simulink model "estimator_designs_main"  (R2022b)
settings: Solver=ode4  StartTime=0.0  StopTime=T  FixedStep=0.002  RelTol=1e-3
values from neighbouring files (symbols this model uses):
  c_lat_f = u(11)    [modelBasedSpeedEstForKalman.m]    (also in validation.m = 140000)
  c_lat_r = u(12)    [modelBasedSpeedEstForKalman.m]    (also in validation.m = 150000)
  c_lon_f = u(9)    [modelBasedSpeedEstForKalman.m]    (also in validation.m = 180000)
  c_lon_r = u(10)    [modelBasedSpeedEstForKalman.m]    (also in validation.m = 200000)
  dt = u(4)    [kinematicVelocity.m]    (also in modelBasedSpeedEstForKalman.m = u(27); validation.m = 0.01)
  eps_bw_acc = 0.1    [validation.m]
  eps_ekf_m_bw_v_u = 0.5    [validation.m]
  eps_m_v = 1    [validation.m]
  m = u(7)    [modelBasedSpeedEstForKalman.m]    (also in validation.m = 3020)
  num_of_signals = 12    [validation.m]
  P0 = diag([1e-5, 1e-5, 1e-5])    [validation.m]
  Q_ekf_1 = diag([1e-5, 1e-2, 1e-2])    [validation.m]
  R = u(9)    [bestWheelSpeedUpdate.m]    (also in modelBasedSpeedEstForKalman.m = u(13); validation.m = 0.3615)
  r_COG_FL = u(10:12)    [bestWheelSpeedUpdate.m]    (also in validation.m = [wheelbase_COG_front; front_track_width / 2; 0])
  r_COG_FR = u(13:15)    [bestWheelSpeedUpdate.m]    (also in validation.m = [wheelbase_COG_front; -front_track_width / 2; 0])
  r_COG_RL = u(16:18)    [bestWheelSpeedUpdate.m]    (also in validation.m = [-wheelbase_COG_rear; rear_track_width / 2; 0])
  r_COG_RR = u(19:21)    [bestWheelSpeedUpdate.m]    (also in validation.m = [-wheelbase_COG_rear; -rear_track_width / 2; 0])
  R_ekf_1 = 1e-2    (= 0.01)    [validation.m]
  sequence_length = 50    [validation.m]
  theta_z = 7145    [validation.m]
  thr_ekf_m_bw_v_u = 5    [validation.m]
  x0 = [0.0001; 0.0001; 0.0001]    [validation.m]
undefined symbols (not defined in the file or in its folder): Discrete, Time
libraries: deeplib x2, ctrlSharedLib x1
(part 1 of 2)
settings Model: Creator=andrzej.skrodzki  LastModifiedBy=andrzej.skrodzki
settings DebuggingCC: SignalInfNanChecking=error  AlgebraicLoopMsg=error  CheckMatrixSingularityMsg=error  IntegerOverflowMsg=error  UnnecessaryDatatypeConvMsg=warning  SignalLabelMismatchMsg=warning  UnconnectedInputMsg=warning  UnconnectedOutputMsg=warning  UnconnectedLineMsg=warning  StrictBusMsg=ErrorOnBusTreatedAsVector  IntegerSaturationMsg=error

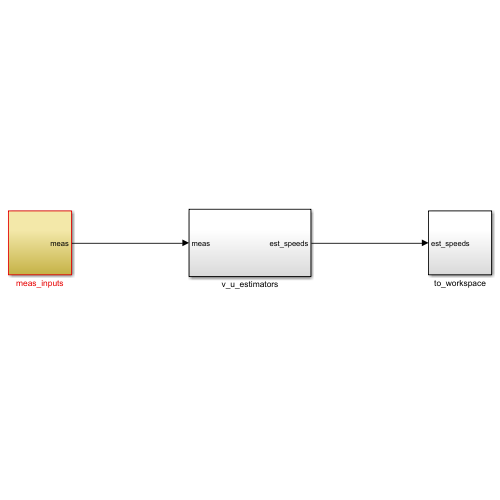
[thumbnail: Simulink's stored preview of the top-level diagram]
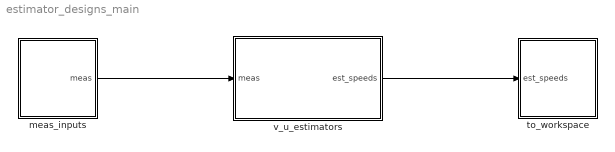
== system estimator_designs_main ==
  meas_inputs : Subsystem
  to_workspace : Subsystem
  v_u_estimators : Subsystem
  wires:
  meas_inputs/1(meas) -> v_u_estimators/1(meas)
  v_u_estimators/1(est_speeds) -> to_workspace/1(est_speeds)

== system estimator_designs_main/meas_inputs ==
  Rate Transition : RateTransition  OutPortSampleTime=0.01
  measurement_replay : Subsystem
  parameters : Subsystem
  sequence_generator : Subsystem
  Bus Element Out : Outport  PortName=meas  Element=SENS_IN_ai_seq_t
  Bus Element Out1 : Outport  PortName=meas  Element=SENS_IN_ai_seq_inf
  Bus Element Out2 : Outport  PortName=meas  Element=SENS_IN
  Bus Element Out3 : Outport  PortName=meas  Element=params
  wires:
  sequence_generator/2(SENS_IN_ai_seq_inf) -> Bus Element Out1/1  "SENS_IN_ai_seq_inf"
  sequence_generator/1(SENS_IN_ai_seq_t) -> Bus Element Out/1  "SENS_IN_ai_seq_t"
  Rate Transition/1 -> Bus Element Out2/1  "SENS_IN"
  measurement_replay/1(SENS_IN) -> Rate Transition/1
  parameters/1(params) -> Bus Element Out3/1

== system estimator_designs_main/to_workspace ==
  BusElementIn : Inport  PortName=est_speeds  Element=v_u_bw
  BusElementIn1 : Inport  PortName=est_speeds  Element=v_u_m
  BusElementIn2 : Inport  PortName=est_speeds  Element=v_u_ekf_m_bw
  BusElementIn3 : Inport  PortName=est_speeds  Element=v_u_ekf_m_ai
  BusElementIn4 : Inport  PortName=est_speeds  Element=veh_u_i7
  BusElementIn5 : Inport  PortName=est_speeds  Element=veh_v
  BusElementIn6 : Inport  PortName=est_speeds  Element=veh_u
  To Workspace : ToWorkspace  VariableName=model_based  SaveFormat=Timeseries  SampleTime=-1
  To Workspace1 : ToWorkspace  VariableName=best_wheel  SaveFormat=Timeseries  SampleTime=-1
  To Workspace2 : ToWorkspace  VariableName=veh_ref  SaveFormat=Timeseries  SampleTime=-1
  To Workspace3 : ToWorkspace  VariableName=ekf_m_bw  SaveFormat=Timeseries  SampleTime=-1
  To Workspace4 : ToWorkspace  VariableName=veh_u  SaveFormat=Timeseries  SampleTime=-1
  To Workspace5 : ToWorkspace  VariableName=veh_v  SaveFormat=Timeseries  SampleTime=-1
  To Workspace6 : ToWorkspace  VariableName=ekf_ai  SaveFormat=Timeseries  SampleTime=-1
  wires:
  BusElementIn4/1 -> To Workspace2/1
  BusElementIn2/1 -> To Workspace3/1
  BusElementIn/1 -> To Workspace1/1
  BusElementIn5/1 -> To Workspace4/1
  BusElementIn3/1 -> To Workspace6/1
  BusElementIn6/1 -> To Workspace5/1
  BusElementIn1/1 -> To Workspace/1

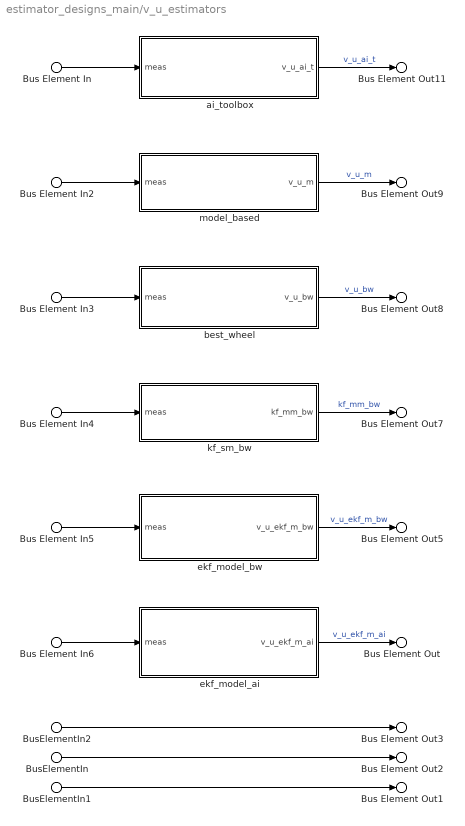
== system estimator_designs_main/v_u_estimators ==
  Bus Element In{,2..6} (6 alike) : Inport  PortName=meas
  BusElementIn : Inport  PortName=meas  Element=SENS_IN.veh_u
  BusElementIn1 : Inport  PortName=meas  Element=SENS_IN.veh_v
  BusElementIn2 : Inport  PortName=meas  Element=SENS_IN.veh_u_i7
  ai_toolbox : Subsystem
  best_wheel : Subsystem
  ekf_model_ai : Subsystem
  ekf_model_bw : Subsystem
  kf_sm_bw : Subsystem
  model_based : Subsystem
  Bus Element Out : Outport  PortName=est_speeds  Element=v_u_ekf_m_ai
  Bus Element Out1 : Outport  PortName=est_speeds  Element=veh_v
  Bus Element Out2 : Outport  PortName=est_speeds  Element=veh_u
  Bus Element Out3 : Outport  PortName=est_speeds  Element=veh_u_i7
  Bus Element Out5 : Outport  PortName=est_speeds  Element=v_u_ekf_m_bw
  Bus Element Out7 : Outport  PortName=est_speeds  Element=v_u_kf_mm_bw
  Bus Element Out8 : Outport  PortName=est_speeds  Element=v_u_bw
  Bus Element Out9 : Outport  PortName=est_speeds  Element=v_u_m
  Bus Element Out11 : Outport  PortName=est_speeds  Element=v_u_ai_t
  wires:
  model_based/1(v_u_m) -> Bus Element Out9/1  "v_u_m"
  best_wheel/1(v_u_bw) -> Bus Element Out8/1  "v_u_bw"
  BusElementIn/1 -> Bus Element Out2/1
  ekf_model_bw/1(v_u_ekf_m_bw) -> Bus Element Out5/1  "v_u_ekf_m_bw"
  ekf_model_ai/1(v_u_ekf_m_ai) -> Bus Element Out/1  "v_u_ekf_m_ai"
  ai_toolbox/1(v_u_ai_t) -> Bus Element Out11/1  "v_u_ai_t"
  kf_sm_bw/1(kf_mm_bw) -> Bus Element Out7/1  "kf_mm_bw"
  BusElementIn1/1 -> Bus Element Out1/1
  BusElementIn2/1 -> Bus Element Out3/1
  Bus Element In/1 -> ai_toolbox/1(meas)
  Bus Element In6/1 -> ekf_model_ai/1(meas)
  Bus Element In5/1 -> ekf_model_bw/1(meas)
  Bus Element In4/1 -> kf_sm_bw/1(meas)
  Bus Element In3/1 -> best_wheel/1(meas)
  Bus Element In2/1 -> model_based/1(meas)

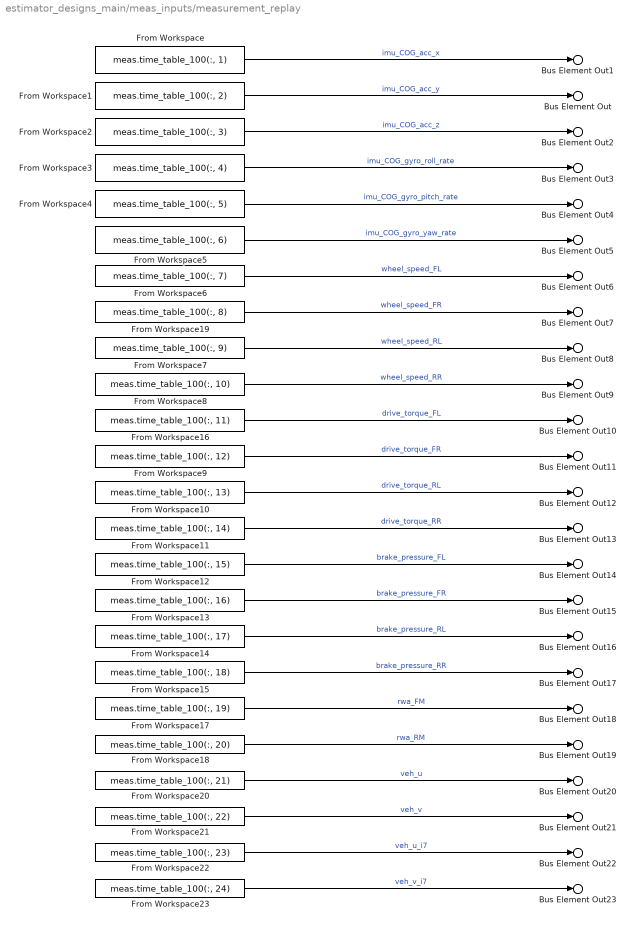
== system estimator_designs_main/meas_inputs/measurement_replay ==
  From Workspace : FromWorkspace  VariableName=meas.time_table_100(:, 1)
  From Workspace1 : FromWorkspace  VariableName=meas.time_table_100(:, 2)
  From Workspace10 : FromWorkspace  VariableName=meas.time_table_100(:, 13)
  From Workspace11 : FromWorkspace  VariableName=meas.time_table_100(:, 14)
  From Workspace12 : FromWorkspace  VariableName=meas.time_table_100(:, 15)
  From Workspace13 : FromWorkspace  VariableName=meas.time_table_100(:, 16)
  From Workspace14 : FromWorkspace  VariableName=meas.time_table_100(:, 17)
  From Workspace15 : FromWorkspace  VariableName=meas.time_table_100(:, 18)
  From Workspace16 : FromWorkspace  VariableName=meas.time_table_100(:, 11)
  From Workspace17 : FromWorkspace  VariableName=meas.time_table_100(:, 19)
  From Workspace18 : FromWorkspace  VariableName=meas.time_table_100(:, 20)
  From Workspace19 : FromWorkspace  VariableName=meas.time_table_100(:, 8)
  From Workspace2 : FromWorkspace  VariableName=meas.time_table_100(:, 3)
  From Workspace20 : FromWorkspace  VariableName=meas.time_table_100(:, 21)
  From Workspace21 : FromWorkspace  VariableName=meas.time_table_100(:, 22)
  From Workspace22 : FromWorkspace  VariableName=meas.time_table_100(:, 23)
  From Workspace23 : FromWorkspace  VariableName=meas.time_table_100(:, 24)
  From Workspace3 : FromWorkspace  VariableName=meas.time_table_100(:, 4)
  From Workspace4 : FromWorkspace  VariableName=meas.time_table_100(:, 5)
  From Workspace5 : FromWorkspace  VariableName=meas.time_table_100(:, 6)
  From Workspace6 : FromWorkspace  VariableName=meas.time_table_100(:, 7)
  From Workspace7 : FromWorkspace  VariableName=meas.time_table_100(:, 9)
  From Workspace8 : FromWorkspace  VariableName=meas.time_table_100(:, 10)
  From Workspace9 : FromWorkspace  VariableName=meas.time_table_100(:, 12)
  Bus Element Out : Outport  PortName=SENS_IN  Element=imu_COG_acc_y
  Bus Element Out1 : Outport  PortName=SENS_IN  Element=imu_COG_acc_x
  Bus Element Out2 : Outport  PortName=SENS_IN  Element=imu_COG_acc_z
  Bus Element Out3 : Outport  PortName=SENS_IN  Element=imu_COG_gyro_roll_rate
  Bus Element Out4 : Outport  PortName=SENS_IN  Element=imu_COG_gyro_pitch_rate
  Bus Element Out5 : Outport  PortName=SENS_IN  Element=imu_COG_gyro_yaw_rate
  Bus Element Out6 : Outport  PortName=SENS_IN  Element=wheel_speed_FL
  Bus Element Out7 : Outport  PortName=SENS_IN  Element=wheel_speed_FR
  Bus Element Out8 : Outport  PortName=SENS_IN  Element=wheel_speed_RL
  Bus Element Out9 : Outport  PortName=SENS_IN  Element=wheel_speed_RR
  Bus Element Out10 : Outport  PortName=SENS_IN  Element=drive_torque_FL
  Bus Element Out11 : Outport  PortName=SENS_IN  Element=drive_torque_FR
  Bus Element Out12 : Outport  PortName=SENS_IN  Element=drive_torque_RL
  Bus Element Out13 : Outport  PortName=SENS_IN  Element=drive_torque_RR
  Bus Element Out14 : Outport  PortName=SENS_IN  Element=brake_pressure_FL
  Bus Element Out15 : Outport  PortName=SENS_IN  Element=brake_pressure_FR
  Bus Element Out16 : Outport  PortName=SENS_IN  Element=brake_pressure_RL
  Bus Element Out17 : Outport  PortName=SENS_IN  Element=brake_pressure_RR
  Bus Element Out18 : Outport  PortName=SENS_IN  Element=rwa_FM
  Bus Element Out19 : Outport  PortName=SENS_IN  Element=rwa_RM
  Bus Element Out20 : Outport  PortName=SENS_IN  Element=veh_u
  Bus Element Out21 : Outport  PortName=SENS_IN  Element=veh_v
  Bus Element Out22 : Outport  PortName=SENS_IN  Element=veh_u_i7
  Bus Element Out23 : Outport  PortName=SENS_IN  Element=veh_v_i7
  wires:
  From Workspace5/1 -> Bus Element Out5/1  "imu_COG_gyro_yaw_rate"
  From Workspace8/1 -> Bus Element Out9/1  "wheel_speed_RR"
  From Workspace17/1 -> Bus Element Out18/1  "rwa_FM"
  From Workspace18/1 -> Bus Element Out19/1  "rwa_RM"
  From Workspace4/1 -> Bus Element Out4/1  "imu_COG_gyro_pitch_rate"
  From Workspace19/1 -> Bus Element Out7/1  "wheel_speed_FR"
  From Workspace6/1 -> Bus Element Out6/1  "wheel_speed_FL"
  From Workspace15/1 -> Bus Element Out17/1  "brake_pressure_RR"
  From Workspace16/1 -> Bus Element Out10/1  "drive_torque_FL"
  From Workspace3/1 -> Bus Element Out3/1  "imu_COG_gyro_roll_rate"
  From Workspace12/1 -> Bus Element Out14/1  "brake_pressure_FL"
  From Workspace2/1 -> Bus Element Out2/1  "imu_COG_acc_z"
  From Workspace10/1 -> Bus Element Out12/1  "drive_torque_RL"
  From Workspace11/1 -> Bus Element Out13/1  "drive_torque_RR"
  From Workspace14/1 -> Bus Element Out16/1  "brake_pressure_RL"
  From Workspace7/1 -> Bus Element Out8/1  "wheel_speed_RL"
  From Workspace13/1 -> Bus Element Out15/1  "brake_pressure_FR"
  From Workspace1/1 -> Bus Element Out/1  "imu_COG_acc_y"
  From Workspace9/1 -> Bus Element Out11/1  "drive_torque_FR"
  From Workspace/1 -> Bus Element Out1/1  "imu_COG_acc_x"
  From Workspace20/1 -> Bus Element Out20/1  "veh_u"
  From Workspace21/1 -> Bus Element Out21/1  "veh_v"
  From Workspace22/1 -> Bus Element Out22/1  "veh_u_i7"
  From Workspace23/1 -> Bus Element Out23/1  "veh_v_i7"

== system estimator_designs_main/meas_inputs/parameters ==
  constants : Subsystem
  Bus Element Out : Outport  PortName=params  Element=m
  Bus Element Out1 : Outport  PortName=params  Element=I_z
  Bus Element Out2 : Outport  PortName=params  Element=C
  Bus Element Out3 : Outport  PortName=params  Element=R
  Bus Element Out4 : Outport  PortName=params  Element=r
  Bus Element Out5 : Outport  PortName=params  Element=eps_m_v
  Bus Element Out6 : Outport  PortName=params  Element=dt
  Bus Element Out7 : Outport  PortName=params  Element=eps_bw_acc
  Bus Element Out8 : Outport  PortName=params  Element=thr_ekf_m_bw_v_u
  Bus Element Out9 : Outport  PortName=params  Element=eps_ekf_m_bw_v_u
  Bus Element Out10 : Outport  PortName=params  Element=R_ekf_1
  Bus Element Out11 : Outport  PortName=params  Element=Q_ekf_1
  wires:
  constants/1(m) -> Bus Element Out/1
  constants/2(I_z) -> Bus Element Out1/1
  constants/3(C) -> Bus Element Out2/1
  constants/4(R) -> Bus Element Out3/1
  constants/5(r) -> Bus Element Out4/1
  constants/6(eps_m_v) -> Bus Element Out5/1
  constants/7(dt) -> Bus Element Out6/1
  constants/8(eps_bw_acc) -> Bus Element Out7/1
  constants/9(thr_ekf_m_bw_v_u) -> Bus Element Out8/1
  constants/10(eps_ekf_m_bw_v_u) -> Bus Element Out9/1
  constants/11(R_ekf_1) -> Bus Element Out10/1
  constants/12(Q_ekf_1) -> Bus Element Out11/1

== system estimator_designs_main/meas_inputs/sequence_generator ==
  Constant1 : Constant  Value=zeros(num_of_signals, sequence_length)
  Constant2 : Constant  Value=zeros(sequence_length, num_of_signals)
  Delay1 : Delay  DelayLength=1  InitialConditionSource=Input port
      settings: InputPortMap=u0,p4
  Delay2 : Delay  DelayLength=1  InitialConditionSource=Input port
      settings: InputPortMap=u0,p4
  MATLAB Function1 : MATLAB Function  TreatAsAtomicUnit=on
  MATLAB Function4 : MATLAB Function  TreatAsAtomicUnit=on
  Rate Transition1 : RateTransition  OutPortSampleTime=0.01
  Reshape : Reshape  OutputDimensionality=Customize  OutputDimensions=[1, sequence_length, num_of_signals]
  Subsystem : Subsystem
  SENS_IN_ai_seq_t : Outport
  SENS_IN_ai_seq_inf : Outport  Port=2
  wires:
  Rate Transition1/1 -> MATLAB Function4/1(SNES_IN_ai), MATLAB Function1/1(SENS_IN_ai)  "SENS_IN_ai"
  Reshape/1 -> SENS_IN_ai_seq_inf/1  "SENS_IN_ai_seq_inf"
  MATLAB Function4/1(SENS_IN_ai_seq) -> Delay2/1, Reshape/1  "SNES_IN_ai_seq_inf"
  Subsystem/1(SENS_IN_ai) -> Rate Transition1/1
  Delay2/1 -> MATLAB Function4/2(SENS_IN_ai_seq_prev)
  Constant2/1 -> Delay2/2
  Constant1/1 -> Delay1/2
  MATLAB Function1/1(SENS_IN_ai_seq) -> SENS_IN_ai_seq_t/1, Delay1/1  "SENS_IN_ai_seq_t"
  Delay1/1 -> MATLAB Function1/2(SENS_IN_ai_seq_prev)

== system estimator_designs_main/v_u_estimators/ai_toolbox ==
  BusElementIn : Inport  PortName=meas  Element=SENS_IN_ai_seq_t
  Reshape : Reshape  Commented=on  OutputDimensionality=Customize  OutputDimensions=[1,sequence_length, num_of_signals]
  "built-in ai " : deeplib/Predict  Network=Network from MAT-file  NetworkFunction=squeezenet  NetworkFilePath=file:///C:/work/0_currently_in_use/AI_training_matlab/trained_models/GRU/trainedGRU.mat  MiniBatchSize=1  InputDataFormats={'',''}  Predictions=on  Activations={}  ForceInterpretedSim=off  EnableDLNetwork=on
  built-in ai 1 : deeplib/Predict  Commented=on  Network=Network from MAT-file  NetworkFunction=squeezenet  NetworkFilePath=file:///C:/work/0_currently_in_use/estimator_designs/models/TCN/it_1/for_matlab/mat/lon/model_TCN_lon 129_conv2d.mat  MiniBatchSize=1  InputDataFormats={ 'input', 'BTC' }  Predictions=on  Activations={}  ForceInterpretedSim=off  EnableDLNetwork=on
  v_u_ai_t : Outport
  wires:
  BusElementIn/1 -> Reshape/1, "built-in ai "/1
  "built-in ai "/1 -> v_u_ai_t/1  "v_u_ai_t"
  built-in ai 1/1 -> ?  "v_u_ai_t"
  Reshape/1 -> built-in ai 1/1

== system estimator_designs_main/v_u_estimators/best_wheel ==
  meas : Inport
  Delay : Delay  DelayLength=1
  best_wheel_speed_est : MATLAB Function  TreatAsAtomicUnit=on
  input_generator : Subsystem
  v_u_bw : Outport
  wires:
  best_wheel_speed_est/1(v_u_bw) -> v_u_bw/1  "v_u_bw"
  meas/1 -> input_generator/1(meas)
  input_generator/1(u) -> best_wheel_speed_est/1(u)
  best_wheel_speed_est/2(sign_acc) -> Delay/1
  Delay/1 -> input_generator/2(prev_sign_acc)

== system estimator_designs_main/v_u_estimators/ekf_model_ai ==
  meas : Inport
  ai_inference_function : Subsystem
  ekf_custom : Subsystem
  input_generator_model : Subsystem
  v_u_ekf_m_ai : Outport
  wires:
  input_generator_model/1(StateTransitionFcnInputs) -> ekf_custom/1(StateTransitionFcnInputs)
  meas/1 -> ekf_custom/3(meas), ai_inference_function/1(meas), input_generator_model/1(meas)
  ai_inference_function/1(v_u_ai_inf) -> ekf_custom/2(v_u_ai_inf)
  ekf_custom/1(v_u_ekf_m_bw) -> v_u_ekf_m_ai/1  "v_u_ekf_m_ai"

== system estimator_designs_main/v_u_estimators/ekf_model_bw ==
  meas : Inport
  ekf_custom : Subsystem
  input_generator_model : Subsystem
  meas_update_bw : Subsystem
  v_u_ekf_m_bw : Outport
  wires:
  meas/1 -> ekf_custom/3(meas), meas_update_bw/1(meas), input_generator_model/1(meas)
  input_generator_model/1(StateTransitionFcnInputs) -> ekf_custom/1(StateTransitionFcnInputs)
  meas_update_bw/1(v_u_bw) -> ekf_custom/2(v_u_bw)
  ekf_custom/1(v_u_ekf_m_bw) -> v_u_ekf_m_bw/1  "v_u_ekf_m_bw"

== system estimator_designs_main/v_u_estimators/kf_sm_bw ==
  meas : Inport
  Selector1 : Selector  InputPortWidth=3  IndexOptions=Index vector (dialog)  Indices=[1]  OutputSizes=1
  Terminator : Terminator
  kf_sm : ctrlSharedLib/Kalman Filter  TimeDomain=Discrete-Time  UseCurrentEstimator=on  ModelSource=Individual A, B, C, D matrices  ModelSourceVariable=ss(0.95,1,1,0,1)  A=diag([1, 0.99, 0.99])  B=0  C=[1,0,0]  D=0  NumberOfStates=1  NumberOfInputs=1  NumberOfOutputs=1  InitialEstimateSource=Dialog  X0=[0;0;0]  P0=10  UseK=off  UseGH=off  NumberOfProcessNoiseInputs=1  G=1  TimeInvariantG=on  H=0  TimeInvariantH=on  Q=diag([0.0025, 0.04, 7.615e-5])  TimeInvariantQ=on  R=0.001  TimeInvariantR=on  N=0  TimeInvariantN=on  AddInputPort=off  AddEnablePort=off  OutputEstimatedY=off  OutputP=off  Ts=-1
  meas_update_ai : Subsystem
  meas_update_bw : Subsystem
  kf_mm_bw : Outport
  wires:
  kf_sm/1 -> Selector1/1
  Selector1/1 -> kf_mm_bw/1
  meas_update_bw/1(v_u_bw) -> kf_sm/1
  meas/1 -> meas_update_ai/1(meas), meas_update_bw/1(meas)
  meas_update_ai/1(v_u_ai_inf) -> Terminator/1

== system estimator_designs_main/v_u_estimators/model_based ==
  meas : Inport
  Delay : Delay  DelayLength=1
  Selector : Selector  InputPortWidth=3  IndexOptions=Index vector (dialog)  Indices=[1]  OutputSizes=1
  input_generator : Subsystem
  model_based_speed_est1 : MATLAB Function  TreatAsAtomicUnit=on
  v_u_m : Outport
  wires:
  model_based_speed_est1/1(x_plus) -> Selector/1, Delay/1  "x_plus"
  Delay/1 -> model_based_speed_est1/1(x)
  meas/1 -> input_generator/1(meas)
  input_generator/1(u) -> model_based_speed_est1/2(u)
  Selector/1 -> v_u_m/1  "v_u_m"

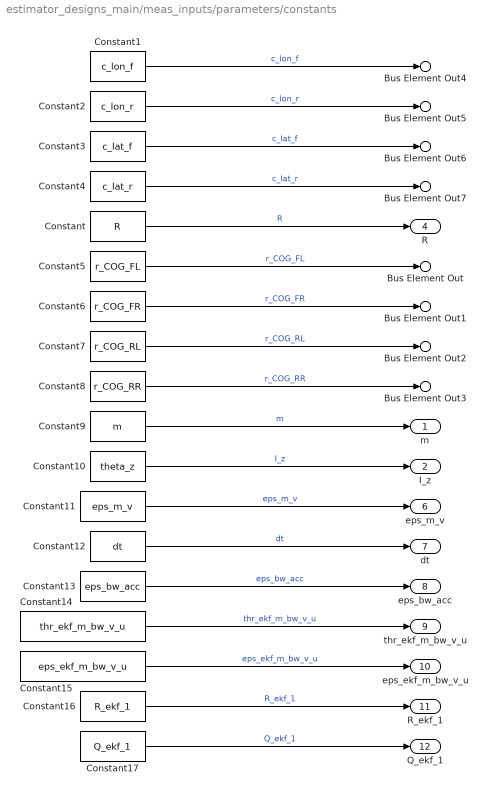
== system estimator_designs_main/meas_inputs/parameters/constants ==
  Constant : Constant  Value=R
  Constant1 : Constant  Value=c_lon_f
  Constant10 : Constant  Value=theta_z
  Constant11 : Constant  Value=eps_m_v
  Constant12 : Constant  Value=dt
  Constant13 : Constant  Value=eps_bw_acc
  Constant14 : Constant  Value=thr_ekf_m_bw_v_u
  Constant15 : Constant  Value=eps_ekf_m_bw_v_u
  Constant16 : Constant  Value=R_ekf_1
  Constant17 : Constant  Value=Q_ekf_1
  Constant2 : Constant  Value=c_lon_r
  Constant3 : Constant  Value=c_lat_f
  Constant4 : Constant  Value=c_lat_r
  Constant5 : Constant  Value=r_COG_FL
  Constant6 : Constant  Value=r_COG_FR
  Constant7 : Constant  Value=r_COG_RL
  Constant8 : Constant  Value=r_COG_RR
  Constant9 : Constant  Value=m
  m : Outport
  I_z : Outport  Port=2
  Bus Element Out4 : Outport  Port=3  PortName=C  Element=c_lon_f
  Bus Element Out5 : Outport  Port=3  PortName=C  Element=c_lon_r
  Bus Element Out6 : Outport  Port=3  PortName=C  Element=c_lat_f
  Bus Element Out7 : Outport  Port=3  PortName=C  Element=c_lat_r
  R : Outport  Port=4
  Bus Element Out : Outport  Port=5  PortName=r  Element=r_COG_FL
  Bus Element Out1 : Outport  Port=5  PortName=r  Element=r_COG_FR
  Bus Element Out2 : Outport  Port=5  PortName=r  Element=r_COG_RL
  Bus Element Out3 : Outport  Port=5  PortName=r  Element=r_COG_RR
  eps_m_v : Outport  Port=6
  dt : Outport  Port=7
  eps_bw_acc : Outport  Port=8
  thr_ekf_m_bw_v_u : Outport  Port=9
  eps_ekf_m_bw_v_u : Outport  Port=10
  R_ekf_1 : Outport  Port=11
  Q_ekf_1 : Outport  Port=12
  wires:
  Constant6/1 -> Bus Element Out1/1  "r_COG_FR"
  Constant3/1 -> Bus Element Out6/1  "c_lat_f"
  Constant4/1 -> Bus Element Out7/1  "c_lat_r"
  Constant/1 -> R/1  "R"
  Constant7/1 -> Bus Element Out2/1  "r_COG_RL"
  Constant1/1 -> Bus Element Out4/1  "c_lon_f"
  Constant5/1 -> Bus Element Out/1  "r_COG_FL"
  Constant8/1 -> Bus Element Out3/1  "r_COG_RR"
  Constant2/1 -> Bus Element Out5/1  "c_lon_r"
  Constant9/1 -> m/1  "m"
  Constant10/1 -> I_z/1  "I_z"
  Constant11/1 -> eps_m_v/1  "eps_m_v"
  Constant12/1 -> dt/1  "dt"
  Constant13/1 -> eps_bw_acc/1  "eps_bw_acc"
  Constant14/1 -> thr_ekf_m_bw_v_u/1  "thr_ekf_m_bw_v_u"
  Constant15/1 -> eps_ekf_m_bw_v_u/1  "eps_ekf_m_bw_v_u"
  Constant16/1 -> R_ekf_1/1  "R_ekf_1"
  Constant17/1 -> Q_ekf_1/1  "Q_ekf_1"

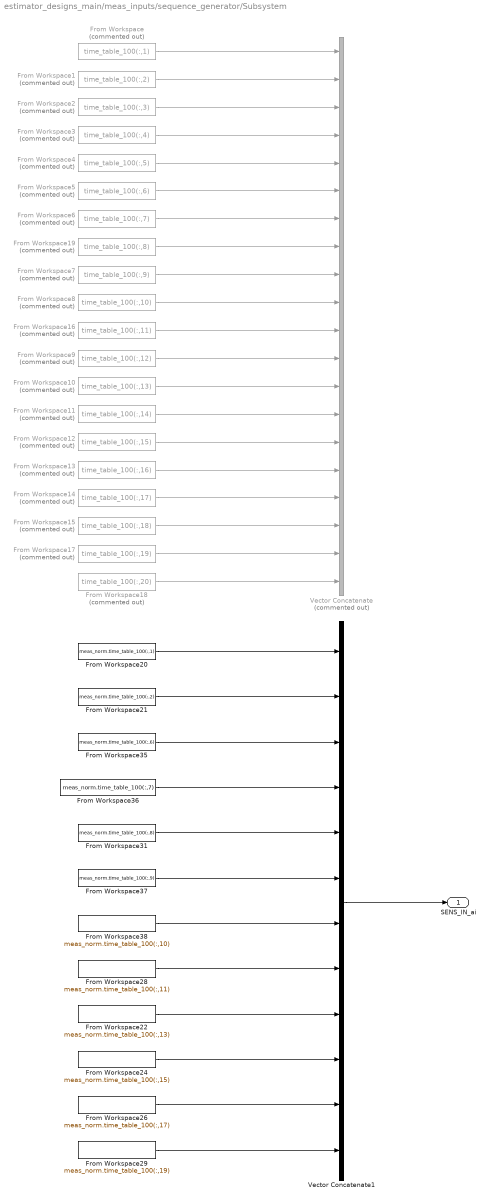
== system estimator_designs_main/meas_inputs/sequence_generator/Subsystem ==
  From Workspace : FromWorkspace  Commented=on  VariableName=time_table_100(:,1)
  From Workspace1 : FromWorkspace  Commented=on  VariableName=time_table_100(:,2)
  From Workspace10 : FromWorkspace  Commented=on  VariableName=time_table_100(:,13)
  From Workspace11 : FromWorkspace  Commented=on  VariableName=time_table_100(:,14)
  From Workspace12 : FromWorkspace  Commented=on  VariableName=time_table_100(:,15)
  From Workspace13 : FromWorkspace  Commented=on  VariableName=time_table_100(:,16)
  From Workspace14 : FromWorkspace  Commented=on  VariableName=time_table_100(:,17)
  From Workspace15 : FromWorkspace  Commented=on  VariableName=time_table_100(:,18)
  From Workspace16 : FromWorkspace  Commented=on  VariableName=time_table_100(:,11)
  From Workspace17 : FromWorkspace  Commented=on  VariableName=time_table_100(:,19)
  From Workspace18 : FromWorkspace  Commented=on  VariableName=time_table_100(:,20)
  From Workspace19 : FromWorkspace  Commented=on  VariableName=time_table_100(:,8)
  From Workspace2 : FromWorkspace  Commented=on  VariableName=time_table_100(:,3)
  From Workspace20 : FromWorkspace  VariableName=meas_norm.time_table_100(:,1)
  From Workspace21 : FromWorkspace  VariableName=meas_norm.time_table_100(:,2)
  From Workspace22 : FromWorkspace  VariableName=meas_norm.time_table_100(:,13)
  From Workspace24 : FromWorkspace  VariableName=meas_norm.time_table_100(:,15)
  From Workspace26 : FromWorkspace  VariableName=meas_norm.time_table_100(:,17)
  From Workspace28 : FromWorkspace  VariableName=meas_norm.time_table_100(:,11)
  From Workspace29 : FromWorkspace  VariableName=meas_norm.time_table_100(:,19)
  From Workspace3 : FromWorkspace  Commented=on  VariableName=time_table_100(:,4)
  From Workspace31 : FromWorkspace  VariableName=meas_norm.time_table_100(:,8)
  From Workspace35 : FromWorkspace  VariableName=meas_norm.time_table_100(:,6)
  From Workspace36 : FromWorkspace  VariableName=meas_norm.time_table_100(:,7)
  From Workspace37 : FromWorkspace  VariableName=meas_norm.time_table_100(:,9)
  From Workspace38 : FromWorkspace  VariableName=meas_norm.time_table_100(:,10)
  From Workspace4 : FromWorkspace  Commented=on  VariableName=time_table_100(:,5)
  From Workspace5 : FromWorkspace  Commented=on  VariableName=time_table_100(:,6)
  From Workspace6 : FromWorkspace  Commented=on  VariableName=time_table_100(:,7)
  From Workspace7 : FromWorkspace  Commented=on  VariableName=time_table_100(:,9)
  From Workspace8 : FromWorkspace  Commented=on  VariableName=time_table_100(:,10)
  From Workspace9 : FromWorkspace  Commented=on  VariableName=time_table_100(:,12)
  Vector Concatenate : Concatenate  Commented=on  NumInputs=20
  Vector Concatenate1 : Concatenate  NumInputs=12
  SENS_IN_ai : Outport
  wires:
  From Workspace31/1 -> Vector Concatenate1/5
  From Workspace35/1 -> Vector Concatenate1/3
  From Workspace29/1 -> Vector Concatenate1/12
  From Workspace36/1 -> Vector Concatenate1/4
  From Workspace28/1 -> Vector Concatenate1/8
  From Workspace38/1 -> Vector Concatenate1/7
  From Workspace24/1 -> Vector Concatenate1/10
  From Workspace22/1 -> Vector Concatenate1/9
  From Workspace26/1 -> Vector Concatenate1/11
  From Workspace37/1 -> Vector Concatenate1/6
  From Workspace20/1 -> Vector Concatenate1/1
  From Workspace21/1 -> Vector Concatenate1/2
  Vector Concatenate1/1 -> SENS_IN_ai/1
  From Workspace/1 -> Vector Concatenate/1
  From Workspace9/1 -> Vector Concatenate/12
  From Workspace1/1 -> Vector Concatenate/2
  From Workspace13/1 -> Vector Concatenate/16
  From Workspace7/1 -> Vector Concatenate/9
  From Workspace14/1 -> Vector Concatenate/17
  From Workspace11/1 -> Vector Concatenate/14
  From Workspace10/1 -> Vector Concatenate/13
  From Workspace2/1 -> Vector Concatenate/3
  From Workspace12/1 -> Vector Concatenate/15
  From Workspace3/1 -> Vector Concatenate/4
  From Workspace16/1 -> Vector Concatenate/11
  From Workspace15/1 -> Vector Concatenate/18
  From Workspace6/1 -> Vector Concatenate/7
  From Workspace19/1 -> Vector Concatenate/8
  From Workspace4/1 -> Vector Concatenate/5
  From Workspace18/1 -> Vector Concatenate/20
  From Workspace17/1 -> Vector Concatenate/19
  From Workspace8/1 -> Vector Concatenate/10
  From Workspace5/1 -> Vector Concatenate/6

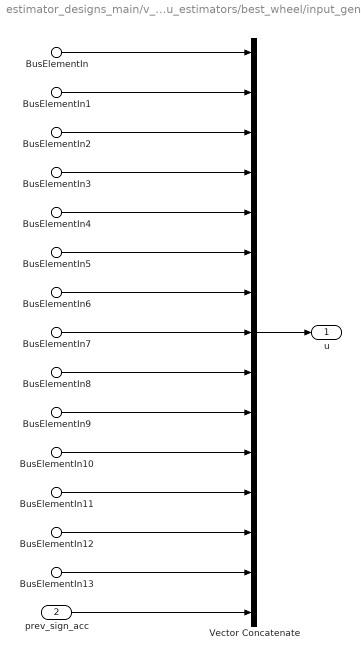
== system estimator_designs_main/v_u_estimators/best_wheel/input_generator ==
  BusElementIn : Inport  PortName=meas  Element=SENS_IN.wheel_speed_FL
  BusElementIn1 : Inport  PortName=meas  Element=SENS_IN.wheel_speed_FR
  BusElementIn2 : Inport  PortName=meas  Element=SENS_IN.wheel_speed_RL
  BusElementIn3 : Inport  PortName=meas  Element=SENS_IN.wheel_speed_RR
  BusElementIn4 : Inport  PortName=meas  Element=SENS_IN.rwa_FM
  BusElementIn5 : Inport  PortName=meas  Element=SENS_IN.rwa_RM
  BusElementIn6 : Inport  PortName=meas  Element=SENS_IN.imu_COG_gyro_yaw_rate
  BusElementIn7 : Inport  PortName=meas  Element=SENS_IN.imu_COG_acc_x
  BusElementIn8 : Inport  PortName=meas  Element=params.R
  BusElementIn9 : Inport  PortName=meas  Element=params.r.r_COG_FL
  BusElementIn10 : Inport  PortName=meas  Element=params.r.r_COG_FR
  BusElementIn11 : Inport  PortName=meas  Element=params.r.r_COG_RL
  BusElementIn12 : Inport  PortName=meas  Element=params.r.r_COG_RR
  BusElementIn13 : Inport  PortName=meas  Element=params.eps_bw_acc
  prev_sign_acc : Inport  Port=2
  Vector Concatenate : Concatenate  NumInputs=15
  u : Outport
  wires:
  Vector Concatenate/1 -> u/1
  BusElementIn/1 -> Vector Concatenate/1
  BusElementIn1/1 -> Vector Concatenate/2
  BusElementIn2/1 -> Vector Concatenate/3
  BusElementIn3/1 -> Vector Concatenate/4
  BusElementIn4/1 -> Vector Concatenate/5
  BusElementIn5/1 -> Vector Concatenate/6
  BusElementIn6/1 -> Vector Concatenate/7
  BusElementIn7/1 -> Vector Concatenate/8
  BusElementIn8/1 -> Vector Concatenate/9
  BusElementIn9/1 -> Vector Concatenate/10
  BusElementIn11/1 -> Vector Concatenate/12
  BusElementIn10/1 -> Vector Concatenate/11
  BusElementIn12/1 -> Vector Concatenate/13
  BusElementIn13/1 -> Vector Concatenate/14
  prev_sign_acc/1 -> Vector Concatenate/15

== system estimator_designs_main/v_u_estimators/ekf_model_ai/ai_inference_function ==
  BusElementIn : Inport  PortName=meas  Element=SENS_IN_ai_seq_inf
  runONNXInference1 : MATLAB Function  TreatAsAtomicUnit=on
  v_u_ai_inf : Outport
  wires:
  BusElementIn/1 -> runONNXInference1/1(inputs)
  runONNXInference1/1(speed_values) -> v_u_ai_inf/1  "v_u_ai_inf"

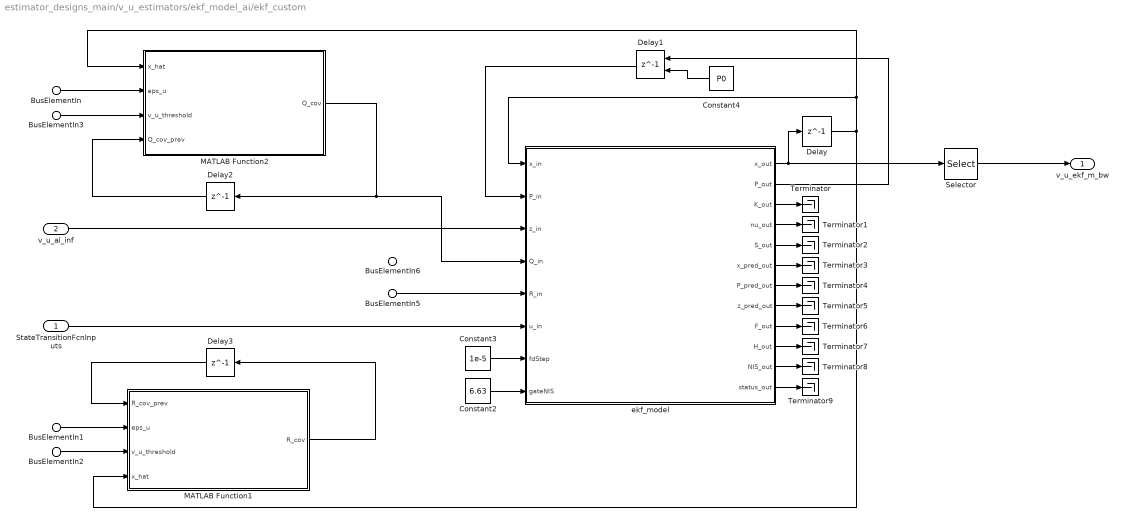
== system estimator_designs_main/v_u_estimators/ekf_model_ai/ekf_custom ==
  StateTransitionFcnInputs : Inport
  v_u_ai_inf : Inport  Port=2
  BusElementIn : Inport  Port=3  PortName=meas  Element=params.eps_ekf_m_bw_v_u
  BusElementIn1 : Inport  Port=3  PortName=meas  Element=params.eps_ekf_m_bw_v_u
  BusElementIn2 : Inport  Port=3  PortName=meas  Element=params.thr_ekf_m_bw_v_u
  BusElementIn3 : Inport  Port=3  PortName=meas  Element=params.thr_ekf_m_bw_v_u
  BusElementIn5 : Inport  Port=3  PortName=meas  Element=params.R_ekf_1
  BusElementIn6 : Inport  Port=3  PortName=meas  Element=params.Q_ekf_1
  Constant2 : Constant  Value=6.63
  Constant3 : Constant  Value=1e-5
  Constant4 : Constant  Value=P0
  Delay : Delay  DelayLength=1  InitialCondition=[0.0001; 0.0001; 0.0001]
  Delay1 : Delay  DelayLength=1  InitialConditionSource=Input port  InitialCondition=diag([1e-10, 1e-10, 1e-10]);
      settings: InputPortMap=u0,p4
  Delay2 : Delay  DelayLength=1
  Delay3 : Delay  DelayLength=1
  MATLAB Function1 : MATLAB Function  TreatAsAtomicUnit=on
  MATLAB Function2 : MATLAB Function  TreatAsAtomicUnit=on
  Selector : Selector  InputPortWidth=3  IndexOptions=Index vector (dialog)  Indices=[1]  OutputSizes=1
  Terminator{,1..9} (10 alike) : Terminator
  ekf_model : MATLAB Function  TreatAsAtomicUnit=on
  v_u_ekf_m_bw : Outport
  wires:
  Selector/1 -> v_u_ekf_m_bw/1
  ekf_model/1(x_out) -> Selector/1, Delay/1
  Delay/1 -> MATLAB Function1/4(x_hat), MATLAB Function2/1(x_hat), ekf_model/1(x_in)
  ekf_model/2(P_out) -> Delay1/1
  Delay1/1 -> ekf_model/2(P_in)
  v_u_ai_inf/1 -> ekf_model/3(z_in)
  StateTransitionFcnInputs/1 -> ekf_model/6(u_in)
  Constant3/1 -> ekf_model/7(fdStep)
  MATLAB Function2/1(Q_cov) -> ekf_model/4(Q_in), Delay2/1
  MATLAB Function1/1(R_cov) -> Delay3/1
  ekf_model/3(K_out) -> Terminator/1
  ekf_model/4(nu_out) -> Terminator1/1
  ekf_model/5(S_out) -> Terminator2/1
  ekf_model/6(x_pred_out) -> Terminator3/1
  ekf_model/7(P_pred_out) -> Terminator4/1
  ekf_model/8(z_pred_out) -> Terminator5/1
  ekf_model/9(F_out) -> Terminator6/1
  ekf_model/10(H_out) -> Terminator7/1
  ekf_model/11(NIS_out) -> Terminator8/1
  ekf_model/12(status_out) -> Terminator9/1
  Constant2/1 -> ekf_model/8(gateNIS)
  Constant4/1 -> Delay1/2
  Delay2/1 -> MATLAB Function2/4(Q_cov_prev)
  Delay3/1 -> MATLAB Function1/1(R_cov_prev)
  BusElementIn/1 -> MATLAB Function2/2(eps_u)
  BusElementIn1/1 -> MATLAB Function1/2(eps_u)
  BusElementIn3/1 -> MATLAB Function2/3(v_u_threshold)
  BusElementIn2/1 -> MATLAB Function1/3(v_u_threshold)
  BusElementIn5/1 -> ekf_model/5(R_in)

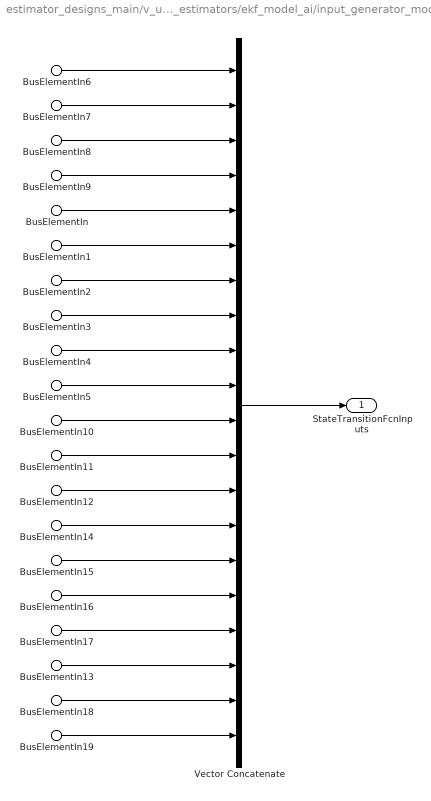
== system estimator_designs_main/v_u_estimators/ekf_model_ai/input_generator_model ==
  BusElementIn6 : Inport  PortName=meas  Element=SENS_IN.wheel_speed_FL
  BusElementIn7 : Inport  PortName=meas  Element=SENS_IN.wheel_speed_FR
  BusElementIn8 : Inport  PortName=meas  Element=SENS_IN.wheel_speed_RL
  BusElementIn9 : Inport  PortName=meas  Element=SENS_IN.wheel_speed_RR
  BusElementIn : Inport  PortName=meas  Element=SENS_IN.rwa_FM
  BusElementIn1 : Inport  PortName=meas  Element=SENS_IN.rwa_RM
  BusElementIn19 : Inport  PortName=meas  Element=SENS_IN.imu_COG_gyro_yaw_rate
  BusElementIn2 : Inport  PortName=meas  Element=params.m
  BusElementIn3 : Inport  PortName=meas  Element=params.I_z
  BusElementIn12 : Inport  PortName=meas  Element=params.R
  BusElementIn13 : Inport  PortName=meas  Element=params.eps_m_v
  BusElementIn14 : Inport  PortName=meas  Element=params.r.r_COG_FL
  BusElementIn15 : Inport  PortName=meas  Element=params.r.r_COG_FR
  BusElementIn16 : Inport  PortName=meas  Element=params.r.r_COG_RL
  BusElementIn17 : Inport  PortName=meas  Element=params.r.r_COG_RR
  BusElementIn18 : Inport  PortName=meas  Element=params.dt
  BusElementIn4 : Inport  PortName=meas  Element=params.C.c_lon_f
  BusElementIn5 : Inport  PortName=meas  Element=params.C.c_lon_r
  BusElementIn10 : Inport  PortName=meas  Element=params.C.c_lat_f
  BusElementIn11 : Inport  PortName=meas  Element=params.C.c_lat_r
  Vector Concatenate : Concatenate  NumInputs=20
  StateTransitionFcnInputs : Outport
  wires:
  Vector Concatenate/1 -> StateTransitionFcnInputs/1
  BusElementIn6/1 -> Vector Concatenate/1
  BusElementIn7/1 -> Vector Concatenate/2
  BusElementIn8/1 -> Vector Concatenate/3
  BusElementIn9/1 -> Vector Concatenate/4
  BusElementIn/1 -> Vector Concatenate/5
  BusElementIn1/1 -> Vector Concatenate/6
  BusElementIn2/1 -> Vector Concatenate/7
  BusElementIn3/1 -> Vector Concatenate/8
  BusElementIn4/1 -> Vector Concatenate/9
  BusElementIn5/1 -> Vector Concatenate/10
  BusElementIn10/1 -> Vector Concatenate/11
  BusElementIn11/1 -> Vector Concatenate/12
  BusElementIn12/1 -> Vector Concatenate/13
  BusElementIn14/1 -> Vector Concatenate/14
  BusElementIn15/1 -> Vector Concatenate/15
  BusElementIn16/1 -> Vector Concatenate/16
  BusElementIn17/1 -> Vector Concatenate/17
  BusElementIn13/1 -> Vector Concatenate/18
  BusElementIn18/1 -> Vector Concatenate/19
  BusElementIn19/1 -> Vector Concatenate/20

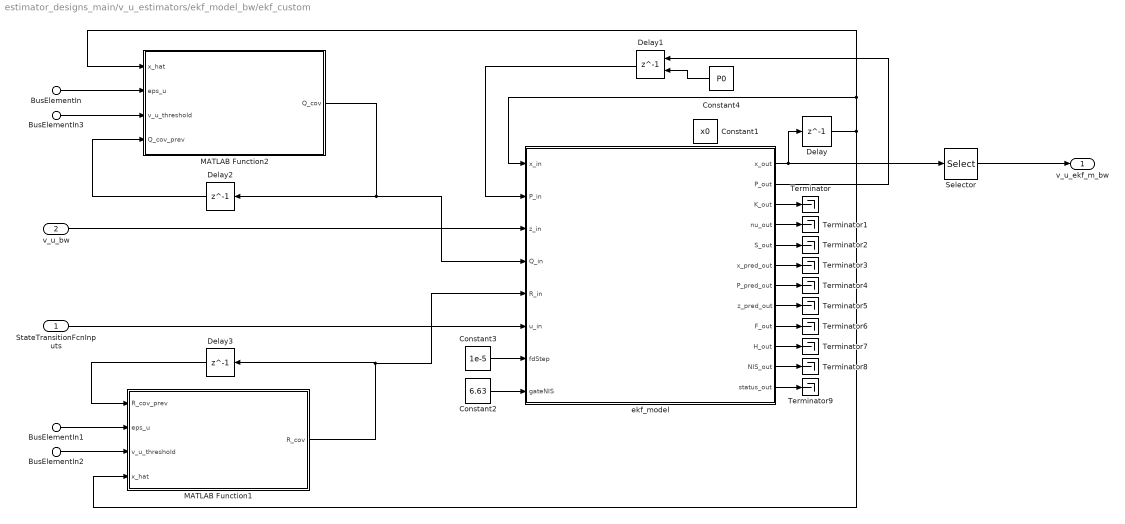
== system estimator_designs_main/v_u_estimators/ekf_model_bw/ekf_custom ==
  StateTransitionFcnInputs : Inport
  v_u_bw : Inport  Port=2
  BusElementIn : Inport  Port=3  PortName=meas  Element=params.eps_ekf_m_bw_v_u
  BusElementIn1 : Inport  Port=3  PortName=meas  Element=params.eps_ekf_m_bw_v_u
  BusElementIn2 : Inport  Port=3  PortName=meas  Element=params.thr_ekf_m_bw_v_u
  BusElementIn3 : Inport  Port=3  PortName=meas  Element=params.thr_ekf_m_bw_v_u
  Constant1 : Constant  Value=x0
  Constant2 : Constant  Value=6.63
  Constant3 : Constant  Value=1e-5
  Constant4 : Constant  Value=P0
  Delay : Delay  DelayLength=1  InitialCondition=[0.0001; 0.0001; 0.0001]
  Delay1 : Delay  DelayLength=1  InitialConditionSource=Input port  InitialCondition=diag([1e-10, 1e-10, 1e-10]);
      settings: InputPortMap=u0,p4
  Delay2 : Delay  DelayLength=1
  Delay3 : Delay  DelayLength=1
  MATLAB Function1 : MATLAB Function  TreatAsAtomicUnit=on
  MATLAB Function2 : MATLAB Function  TreatAsAtomicUnit=on
  Selector : Selector  InputPortWidth=3  IndexOptions=Index vector (dialog)  Indices=[1]  OutputSizes=1
  Terminator{,1..9} (10 alike) : Terminator
  ekf_model : MATLAB Function  TreatAsAtomicUnit=on
  v_u_ekf_m_bw : Outport
  wires:
  Selector/1 -> v_u_ekf_m_bw/1
  ekf_model/1(x_out) -> Selector/1, Delay/1
  Delay/1 -> MATLAB Function1/4(x_hat), MATLAB Function2/1(x_hat), ekf_model/1(x_in)
  ekf_model/2(P_out) -> Delay1/1
  Delay1/1 -> ekf_model/2(P_in)
  v_u_bw/1 -> ekf_model/3(z_in)
  StateTransitionFcnInputs/1 -> ekf_model/6(u_in)
  Constant3/1 -> ekf_model/7(fdStep)
  MATLAB Function2/1(Q_cov) -> ekf_model/4(Q_in), Delay2/1
  MATLAB Function1/1(R_cov) -> ekf_model/5(R_in), Delay3/1
  ekf_model/3(K_out) -> Terminator/1
  ekf_model/4(nu_out) -> Terminator1/1
  ekf_model/5(S_out) -> Terminator2/1
  ekf_model/6(x_pred_out) -> Terminator3/1
  ekf_model/7(P_pred_out) -> Terminator4/1
  ekf_model/8(z_pred_out) -> Terminator5/1
  ekf_model/9(F_out) -> Terminator6/1
  ekf_model/10(H_out) -> Terminator7/1
  ekf_model/11(NIS_out) -> Terminator8/1
  ekf_model/12(status_out) -> Terminator9/1
  Constant2/1 -> ekf_model/8(gateNIS)
  Constant4/1 -> Delay1/2
  Delay2/1 -> MATLAB Function2/4(Q_cov_prev)
  Delay3/1 -> MATLAB Function1/1(R_cov_prev)
  BusElementIn/1 -> MATLAB Function2/2(eps_u)
  BusElementIn1/1 -> MATLAB Function1/2(eps_u)
  BusElementIn3/1 -> MATLAB Function2/3(v_u_threshold)
  BusElementIn2/1 -> MATLAB Function1/3(v_u_threshold)

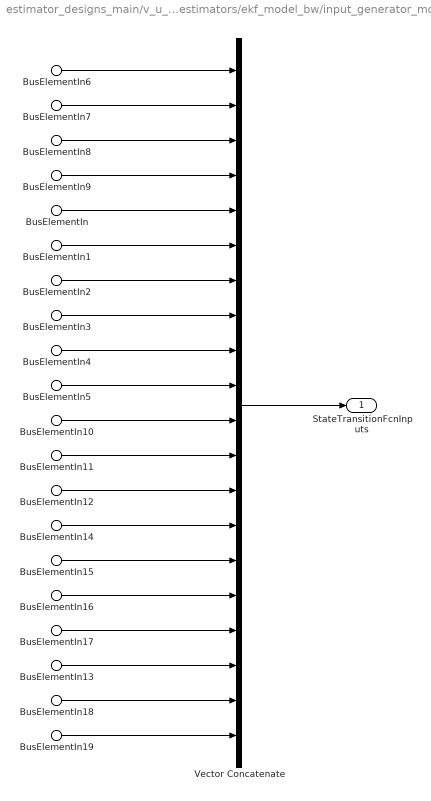
== system estimator_designs_main/v_u_estimators/ekf_model_bw/input_generator_model ==
  BusElementIn6 : Inport  PortName=meas  Element=SENS_IN.wheel_speed_FL
  BusElementIn7 : Inport  PortName=meas  Element=SENS_IN.wheel_speed_FR
  BusElementIn8 : Inport  PortName=meas  Element=SENS_IN.wheel_speed_RL
  BusElementIn9 : Inport  PortName=meas  Element=SENS_IN.wheel_speed_RR
  BusElementIn : Inport  PortName=meas  Element=SENS_IN.rwa_FM
  BusElementIn1 : Inport  PortName=meas  Element=SENS_IN.rwa_RM
  BusElementIn19 : Inport  PortName=meas  Element=SENS_IN.imu_COG_gyro_yaw_rate
  BusElementIn2 : Inport  PortName=meas  Element=params.m
  BusElementIn3 : Inport  PortName=meas  Element=params.I_z
  BusElementIn12 : Inport  PortName=meas  Element=params.R
  BusElementIn13 : Inport  PortName=meas  Element=params.eps_m_v
  BusElementIn14 : Inport  PortName=meas  Element=params.r.r_COG_FL
  BusElementIn15 : Inport  PortName=meas  Element=params.r.r_COG_FR
  BusElementIn16 : Inport  PortName=meas  Element=params.r.r_COG_RL
  BusElementIn17 : Inport  PortName=meas  Element=params.r.r_COG_RR
  BusElementIn18 : Inport  PortName=meas  Element=params.dt
  BusElementIn4 : Inport  PortName=meas  Element=params.C.c_lon_f
  BusElementIn5 : Inport  PortName=meas  Element=params.C.c_lon_r
  BusElementIn10 : Inport  PortName=meas  Element=params.C.c_lat_f
  BusElementIn11 : Inport  PortName=meas  Element=params.C.c_lat_r
  Vector Concatenate : Concatenate  NumInputs=20
  StateTransitionFcnInputs : Outport
  wires:
  Vector Concatenate/1 -> StateTransitionFcnInputs/1
  BusElementIn6/1 -> Vector Concatenate/1
  BusElementIn7/1 -> Vector Concatenate/2
  BusElementIn8/1 -> Vector Concatenate/3
  BusElementIn9/1 -> Vector Concatenate/4
  BusElementIn/1 -> Vector Concatenate/5
  BusElementIn1/1 -> Vector Concatenate/6
  BusElementIn2/1 -> Vector Concatenate/7
  BusElementIn3/1 -> Vector Concatenate/8
  BusElementIn4/1 -> Vector Concatenate/9
  BusElementIn5/1 -> Vector Concatenate/10
  BusElementIn10/1 -> Vector Concatenate/11
  BusElementIn11/1 -> Vector Concatenate/12
  BusElementIn12/1 -> Vector Concatenate/13
  BusElementIn14/1 -> Vector Concatenate/14
  BusElementIn15/1 -> Vector Concatenate/15
  BusElementIn16/1 -> Vector Concatenate/16
  BusElementIn17/1 -> Vector Concatenate/17
  BusElementIn13/1 -> Vector Concatenate/18
  BusElementIn18/1 -> Vector Concatenate/19
  BusElementIn19/1 -> Vector Concatenate/20

== system estimator_designs_main/v_u_estimators/ekf_model_bw/meas_update_bw ==
  meas : Inport
  Delay : Delay  DelayLength=1
  best_wheel_speed_est : MATLAB Function  TreatAsAtomicUnit=on
  input_generator : Subsystem
  v_u_bw : Outport
  wires:
  input_generator/1(u) -> best_wheel_speed_est/1(u)
  best_wheel_speed_est/2(sign_acc) -> Delay/1
  best_wheel_speed_est/1(v_u_bw) -> v_u_bw/1
  Delay/1 -> input_generator/2(prev_sign_acc)
  meas/1 -> input_generator/1(meas)

== system estimator_designs_main/v_u_estimators/kf_sm_bw/meas_update_ai ==
  BusElementIn : Inport  PortName=meas  Element=SENS_IN_ai_seq_inf
  runONNXInference1 : MATLAB Function  TreatAsAtomicUnit=on
  v_u_ai_inf : Outport
  wires:
  BusElementIn/1 -> runONNXInference1/1(inputs)
  runONNXInference1/1(speed_values) -> v_u_ai_inf/1  "v_u_ai_inf"

== system estimator_designs_main/v_u_estimators/kf_sm_bw/meas_update_bw ==
  meas : Inport
  Delay : Delay  DelayLength=1
  best_wheel_speed_est : MATLAB Function  TreatAsAtomicUnit=on
  input_generator : Subsystem
  v_u_bw : Outport
  wires:
  input_generator/1(u) -> best_wheel_speed_est/1(u)
  best_wheel_speed_est/2(sign_acc) -> Delay/1
  best_wheel_speed_est/1(v_u_bw) -> v_u_bw/1
  Delay/1 -> input_generator/2(prev_sign_acc)
  meas/1 -> input_generator/1(meas)

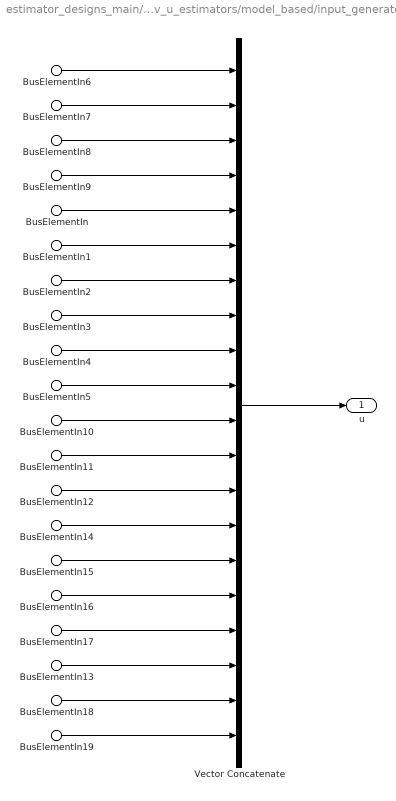
== system estimator_designs_main/v_u_estimators/model_based/input_generator ==
  BusElementIn6 : Inport  PortName=meas  Element=SENS_IN.wheel_speed_FL
  BusElementIn7 : Inport  PortName=meas  Element=SENS_IN.wheel_speed_FR
  BusElementIn8 : Inport  PortName=meas  Element=SENS_IN.wheel_speed_RL
  BusElementIn9 : Inport  PortName=meas  Element=SENS_IN.wheel_speed_RR
  BusElementIn : Inport  PortName=meas  Element=SENS_IN.rwa_FM
  BusElementIn1 : Inport  PortName=meas  Element=SENS_IN.rwa_RM
  BusElementIn19 : Inport  PortName=meas  Element=SENS_IN.imu_COG_gyro_yaw_rate
  BusElementIn2 : Inport  PortName=meas  Element=params.m
  BusElementIn3 : Inport  PortName=meas  Element=params.I_z
  BusElementIn12 : Inport  PortName=meas  Element=params.R
  BusElementIn13 : Inport  PortName=meas  Element=params.eps_m_v
  BusElementIn14 : Inport  PortName=meas  Element=params.r.r_COG_FL
  BusElementIn15 : Inport  PortName=meas  Element=params.r.r_COG_FR
  BusElementIn16 : Inport  PortName=meas  Element=params.r.r_COG_RL
  BusElementIn17 : Inport  PortName=meas  Element=params.r.r_COG_RR
  BusElementIn18 : Inport  PortName=meas  Element=params.dt
  BusElementIn4 : Inport  PortName=meas  Element=params.C.c_lon_f
  BusElementIn5 : Inport  PortName=meas  Element=params.C.c_lon_r
  BusElementIn10 : Inport  PortName=meas  Element=params.C.c_lat_f
  BusElementIn11 : Inport  PortName=meas  Element=params.C.c_lat_r
  Vector Concatenate : Concatenate  NumInputs=20
  u : Outport
  wires:
  Vector Concatenate/1 -> u/1
  BusElementIn6/1 -> Vector Concatenate/1
  BusElementIn7/1 -> Vector Concatenate/2
  BusElementIn8/1 -> Vector Concatenate/3
  BusElementIn9/1 -> Vector Concatenate/4
  BusElementIn/1 -> Vector Concatenate/5
  BusElementIn1/1 -> Vector Concatenate/6
  BusElementIn2/1 -> Vector Concatenate/7
  BusElementIn3/1 -> Vector Concatenate/8
  BusElementIn4/1 -> Vector Concatenate/9
  BusElementIn5/1 -> Vector Concatenate/10
  BusElementIn10/1 -> Vector Concatenate/11
  BusElementIn11/1 -> Vector Concatenate/12
  BusElementIn12/1 -> Vector Concatenate/13
  BusElementIn14/1 -> Vector Concatenate/14
  BusElementIn15/1 -> Vector Concatenate/15
  BusElementIn16/1 -> Vector Concatenate/16
  BusElementIn17/1 -> Vector Concatenate/17
  BusElementIn13/1 -> Vector Concatenate/18
  BusElementIn18/1 -> Vector Concatenate/19
  BusElementIn19/1 -> Vector Concatenate/20

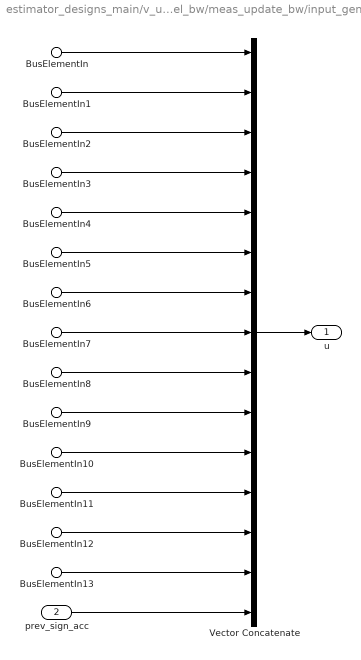
== system estimator_designs_main/v_u_estimators/ekf_model_bw/meas_update_bw/input_generator ==
  BusElementIn : Inport  PortName=meas  Element=SENS_IN.wheel_speed_FL
  BusElementIn1 : Inport  PortName=meas  Element=SENS_IN.wheel_speed_FR
  BusElementIn2 : Inport  PortName=meas  Element=SENS_IN.wheel_speed_RL
  BusElementIn3 : Inport  PortName=meas  Element=SENS_IN.wheel_speed_RR
  BusElementIn4 : Inport  PortName=meas  Element=SENS_IN.rwa_FM
  BusElementIn5 : Inport  PortName=meas  Element=SENS_IN.rwa_RM
  BusElementIn6 : Inport  PortName=meas  Element=SENS_IN.imu_COG_gyro_yaw_rate
  BusElementIn7 : Inport  PortName=meas  Element=SENS_IN.imu_COG_acc_x
  BusElementIn8 : Inport  PortName=meas  Element=params.R
  BusElementIn9 : Inport  PortName=meas  Element=params.r.r_COG_FL
  BusElementIn10 : Inport  PortName=meas  Element=params.r.r_COG_FR
  BusElementIn11 : Inport  PortName=meas  Element=params.r.r_COG_RL
  BusElementIn12 : Inport  PortName=meas  Element=params.r.r_COG_RR
  BusElementIn13 : Inport  PortName=meas  Element=params.eps_bw_acc
  prev_sign_acc : Inport  Port=2
  Vector Concatenate : Concatenate  NumInputs=15
  u : Outport
  wires:
  Vector Concatenate/1 -> u/1
  BusElementIn/1 -> Vector Concatenate/1
  BusElementIn1/1 -> Vector Concatenate/2
  BusElementIn2/1 -> Vector Concatenate/3
  BusElementIn3/1 -> Vector Concatenate/4
  BusElementIn4/1 -> Vector Concatenate/5
  BusElementIn5/1 -> Vector Concatenate/6
  BusElementIn6/1 -> Vector Concatenate/7
  BusElementIn7/1 -> Vector Concatenate/8
  BusElementIn8/1 -> Vector Concatenate/9
  BusElementIn9/1 -> Vector Concatenate/10
  BusElementIn11/1 -> Vector Concatenate/12
  BusElementIn10/1 -> Vector Concatenate/11
  BusElementIn12/1 -> Vector Concatenate/13
  BusElementIn13/1 -> Vector Concatenate/14
  prev_sign_acc/1 -> Vector Concatenate/15

== system estimator_designs_main/v_u_estimators/kf_sm_bw/meas_update_bw/input_generator ==
  BusElementIn : Inport  PortName=meas  Element=SENS_IN.wheel_speed_FL
  BusElementIn1 : Inport  PortName=meas  Element=SENS_IN.wheel_speed_FR
  BusElementIn2 : Inport  PortName=meas  Element=SENS_IN.wheel_speed_RL
  BusElementIn3 : Inport  PortName=meas  Element=SENS_IN.wheel_speed_RR
  BusElementIn4 : Inport  PortName=meas  Element=SENS_IN.rwa_FM
  BusElementIn5 : Inport  PortName=meas  Element=SENS_IN.rwa_RM
  BusElementIn6 : Inport  PortName=meas  Element=SENS_IN.imu_COG_gyro_yaw_rate
  BusElementIn7 : Inport  PortName=meas  Element=SENS_IN.imu_COG_acc_x
  BusElementIn8 : Inport  PortName=meas  Element=params.R
  BusElementIn9 : Inport  PortName=meas  Element=params.r.r_COG_FL
  BusElementIn10 : Inport  PortName=meas  Element=params.r.r_COG_FR
  BusElementIn11 : Inport  PortName=meas  Element=params.r.r_COG_RL
  BusElementIn12 : Inport  PortName=meas  Element=params.r.r_COG_RR
  BusElementIn13 : Inport  PortName=meas  Element=params.eps_bw_acc
  prev_sign_acc : Inport  Port=2
  Vector Concatenate : Concatenate  NumInputs=15
  u : Outport
  wires:
  Vector Concatenate/1 -> u/1
  BusElementIn/1 -> Vector Concatenate/1
  BusElementIn1/1 -> Vector Concatenate/2
  BusElementIn2/1 -> Vector Concatenate/3
  BusElementIn3/1 -> Vector Concatenate/4
  BusElementIn4/1 -> Vector Concatenate/5
  BusElementIn5/1 -> Vector Concatenate/6
  BusElementIn6/1 -> Vector Concatenate/7
  BusElementIn7/1 -> Vector Concatenate/8
  BusElementIn8/1 -> Vector Concatenate/9
  BusElementIn9/1 -> Vector Concatenate/10
  BusElementIn11/1 -> Vector Concatenate/12
  BusElementIn10/1 -> Vector Concatenate/11
  BusElementIn12/1 -> Vector Concatenate/13
  BusElementIn13/1 -> Vector Concatenate/14
  prev_sign_acc/1 -> Vector Concatenate/15

== matlab function estimator_designs_main/v_u_estimators/model_based/model_based_speed_est1 ==
  data: x input size=3; x_plus output size=3; u input size=28
function x_plus  = modelBasedSpeedEst(x, u)

% assigning the inputs

% time varying inputs
omega_w_FL = u(1);
omega_w_FR = u(2);
omega_w_RL = u(3);
omega_w_RR = u(4);

delta_FL = u(5);
delta_FR = u(5);
delta_RL = u(6);
delta_RR = u(6);

% parameter inputs
m = u(7);
I_z = u(8);

c_lon_f = u(9);
c_lon_r = u(10);
c_lat_f = u(11);
c_lat_r = u(12);

R = u(13);

% COG -> tire
r_FL = u(14:16);
r_FR = u(17:19);
r_RL = u(20:22);
r_RR = u(23:25);

eps_v_u = u(26);

dt = u(27);

% w_z = u(28);

% assigning the state variables

v_x = x(1);
v_y = x(2);
w_z = x(3);

% to avoid 0 division
if v_x <= 0.5
    v_x = 0.5;   
end

v = [v_x; v_y; 0];
w = [0; 0; w_z];

% transformation matrices
T_FL = [cos(delta_FL), sin(delta_FL), 0; -sin(delta_FL), cos(delta_FL), 0; 0, 0, 1];
T_FL_neg = [cos(-delta_FL), sin(-delta_FL), 0; -sin(-delta_FL), cos(-delta_FL), 0; 0, 0, 1];

T_FR = [cos(delta_FR), sin(delta_FR), 0; -sin(delta_FR), cos(delta_FR), 0; 0, 0, 1];
T_FR_neg = [cos(-delta_FR), sin(-delta_FR), 0; -sin(-delta_FR), cos(-delta_FR), 0; 0, 0, 1];

T_RL = [cos(delta_RL), sin(delta_RL), 0; -sin(delta_RL), cos(delta_RL), 0; 0, 0, 1];
T_RL_neg = [cos(-delta_RL), sin(-delta_RL), 0; -sin(-delta_RL), cos(-delta_RL), 0; 0, 0, 1];

T_RR = [cos(delta_RR), sin(delta_RR), 0; -sin(delta_RR), cos(delta_RR), 0; 0, 0, 1];
T_RR_neg = [cos(-delta_RR), sin(-delta_RR), 0; -sin(-delta_RR), cos(-delta_RR), 0; 0, 0, 1];

% wheel velocity (in the wheel coordinate system) from the vehicle velocity

v_w_FL = T_FL*(v + cross(w, r_FL));
v_w_FR = T_FR*(v + cross(w, r_FR));
v_w_RL = T_RL*(v + cross(w, r_RL));
v_w_RR = T_RR*(v + cross(w, r_RR));

v_w = [v_w_FL, v_w_FR, v_w_RL, v_w_RR];

% Longitdunal slip and sideslip angle calculation

% Denominators (robust to near-zero or sign changes)
den_FL = max(eps_v_u, abs(v_w(1,1)));
den_FR = max(eps_v_u, abs(v_w(1,2)));
den_RL = max(eps_v_u, abs(v_w(1,3)));
den_RR = max(eps_v_u, abs(v_w(1,4)));

% Longitudinal slip
k_FL = -(v_w(1,1) - omega_w_FL*R) / den_FL;
k_FR = -(v_w(1,2) - omega_w_FR*R) / den_FR;
k_RL = -(v_w(1,3) - omega_w_RL*R) / den_RL;
k_RR = -(v_w(1,4) - omega_w_RR*R) / den_RR;

k = [k_FL; k_FR; k_RL; k_RR];

% Lateral side slip angles

alfa_FL = atan2(-v_w(2,1), den_FL);
alfa_FR = atan2(-v_w(2,2), den_FR);
alfa_RL = atan2(-v_w(2,3), den_RL);
alfa_RR = atan2(-v_w(2,4), den_RR);

alfa = [alfa_FL; alfa_FR; alfa_RL; alfa_RR];

% tire forces
F_t_FL_x = k(1) * c_lon_f;
F_t_FR_x = k(2) * c_lon_f;
F_t_RL_x = k(3) * c_lon_r;
F_t_RR_x = k(4) * c_lon_r;

F_t_FL_y = alfa(1) * c_lat_f;
F_t_FR_y = alfa(2) * c_lat_f;
F_t_RL_y = alfa(3) * c_lat_r;
F_t_RR_y = alfa(4) * c_lat_r;

F_t_FL = [F_t_FL_x; F_t_FL_y; 0];
F_t_FR = [F_t_FR_x; F_t_FR_y; 0];
F_t_RL = [F_t_RL_x; F_t_RL_y; 0];
F_t_RR = [F_t_RR_x; F_t_RR_y; 0];

% expressing the COG force and torque
F_t_FL_T = T_FL_neg * F_t_FL;
F_t_FR_T = T_FR_neg * F_t_FR;
F_t_RL_T = T_RL_neg * F_t_RL;
F_t_RR_T = T_RR_neg * F_t_RR;

F_COG = F_t_FL_T + F_t_FR_T + F_t_RL_T + F_t_RR_T;

M_COG = cross(r_FL, F_t_FL_T) + cross(r_FR, F_t_FR_T) + cross(r_RL, F_t_RL_T) + cross(r_RR, F_t_RR_T);

% expressing v_x_dot, v_y_dot and w_z_dot
v_x_dot = F_COG(1)/m + w(3)*v(2);

v_y_dot = F_COG(2)/m - w(3)*v(1);

w_dot = M_COG / I_z;

w_z_dot = w_dot(3);

% forward Euler method for the next step's values

v_x_plus = v_x_dot * dt + v_x;
v_y_plus = v_y_dot * dt + v_y;
w_z_plus = w_z_dot * dt + w_z;

% if v_x_plus < 0
%     v_x_plus = 0;
% end

x_plus = [v_x_plus; v_y_plus; w_z_plus];

end
